simulink subsystem "Day1_Scenario_2"  (R2024a)
settings: Solver=VariableStepAuto  StartTime=0.0  StopTime=10.0  RelTol=1e-3
libraries: CarMaker4SL x2
settings Model: Creator=junhyung.cha  LastModifiedBy=User

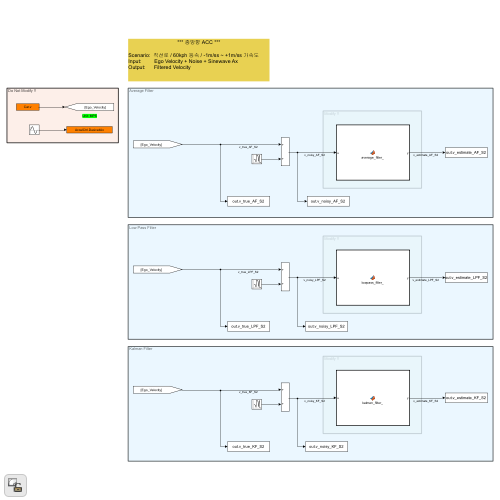
[thumbnail: Simulink's stored preview of the top-level diagram]
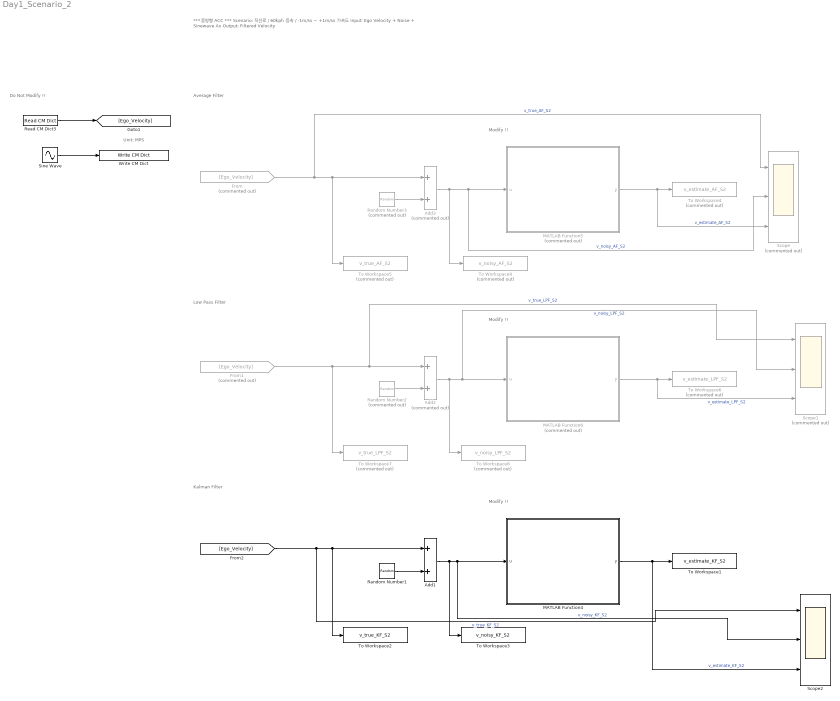
== system Day1_Scenario_2 ==
  note: Do Not Modify !!
  note: Low Pass Filter
  note: Average Filter
  note: Modify !!
  note: Modify !!
  note: Kalman Filter
  note: Modify !!
  note: *** 종방향 ACC ***
      |
      | Scenario: 직선로 / 60kph 등속 / -1m/ss ~ +1m/ss 가속도
      | Input: Ego Velocity + Noise + Sinewave Ax
      | Output: Filtered Velocity
  note: Unit: MPS
  Add1 : Sum
  Add2 : Sum  Commented=on
  Add3 : Sum  Commented=on
  From : From  Commented=on  GotoTag=Ego_Velocity
  From1 : From  Commented=on  GotoTag=Ego_Velocity
  MATLAB Function4 : MATLAB Function  TreatAsAtomicUnit=on
  MATLAB Function5 : MATLAB Function  Commented=on  TreatAsAtomicUnit=on
  MATLAB Function6 : MATLAB Function  Commented=on  TreatAsAtomicUnit=on
  Random Number1 : RandomNumber
  Random Number2 : RandomNumber  Commented=on
  Random Number3 : RandomNumber  Commented=on
  Read CM Dict3 : CarMaker4SL/Read CM Dict  xname=Car.v  xsync=off  xstime=Inherited
  Scope : Scope  Commented=on  NumInputPorts=3
  Scope1 : Scope  Commented=on  NumInputPorts=3
  Scope2 : Scope  NumInputPorts=3
  Sine Wave : Sin
  To Workspace1 : ToWorkspace  VariableName=v_estimate_KF_S2  SaveFormat=Timeseries  SampleTime=-1
  To Workspace2 : ToWorkspace  VariableName=v_true_KF_S2  SaveFormat=Timeseries  SampleTime=-1
  To Workspace3 : ToWorkspace  VariableName=v_noisy_KF_S2  SaveFormat=Timeseries  SampleTime=-1
  To Workspace4 : ToWorkspace  Commented=on  VariableName=v_estimate_AF_S2  SaveFormat=Timeseries  SampleTime=-1
  To Workspace5 : ToWorkspace  Commented=on  VariableName=v_true_AF_S2  SaveFormat=Timeseries  SampleTime=-1
  To Workspace6 : ToWorkspace  Commented=on  VariableName=v_estimate_LPF_S2  SaveFormat=Timeseries  SampleTime=-1
  To Workspace7 : ToWorkspace  Commented=on  VariableName=v_true_LPF_S2  SaveFormat=Timeseries  SampleTime=-1
  To Workspace8 : ToWorkspace  Commented=on  VariableName=v_noisy_LPF_S2  SaveFormat=Timeseries  SampleTime=-1
  To Workspace9 : ToWorkspace  Commented=on  VariableName=v_noisy_AF_S2  SaveFormat=Timeseries  SampleTime=-1
  Write CM Dict : CarMaker4SL/Write CM Dict  xname=AccelCtrl.DesiredAx  xsync=off
  wires:
  Sine Wave/1 -> Write CM Dict/1
  Random Number3/1 -> Add3/2
  Add3/1 -> To Workspace9/1, MATLAB Function5/1(u), Scope/2  "v_noisy_AF_S2"
  Add2/1 -> To Workspace8/1, MATLAB Function6/1(u), Scope1/2  "v_noisy_LPF_S2"
  From1/1 -> Add2/1, Scope1/1, To Workspace7/1  "v_true_LPF_S2"
  MATLAB Function6/1(y) -> To Workspace6/1, Scope1/3  "v_estimate_LPF_S2"
  Random Number2/1 -> Add2/2
  MATLAB Function5/1(y) -> To Workspace4/1, Scope/3  "v_estimate_AF_S2"
  Add1/1 -> To Workspace3/1, MATLAB Function4/1(u), Scope2/2  "v_noisy_KF_S2"
  [Ego_Velocity] -> Add1/1, To Workspace2/1, Scope2/1  "v_true_KF_S2"
  MATLAB Function4/1(y) -> To Workspace1/1, Scope2/3  "v_estimate_KF_S2"
  From/1 -> Add3/1, To Workspace5/1, Scope/1  "v_true_AF_S2"
  Random Number1/1 -> Add1/2
  Read CM Dict3/1 -> [Ego_Velocity]

== matlab function Day1_Scenario_2/MATLAB Function5 ==
  settings: updateMethod=DISCRETE  sampleTime=0.05
  data: u input; y output
% function y = average_filter_(u)
%     y = 0;
% end


function y = average_filter_(u)
% 평균 필터 (5포인트 이동 평균)
% 입력: u - 현재 noisy 값
% 출력: y - 평균 필터된 값

persistent buffer
persistent idx
persistent count

N = 5; % 평균을 낼 샘플 수 (필터 윈도우 크기)

if isempty(buffer)
    buffer = zeros(1, N);
    idx = 1;
    count = 0;
end

% 새로운 값 저장
buffer(idx) = u;
idx = idx + 1;
if idx > N
    idx = 1;
end

% 현재까지 받은 값 수 증가
if count < N
    count = count + 1;
end

% 평균 계산
y = sum(buffer) / count;

== matlab function Day1_Scenario_2/MATLAB Function6 ==
  settings: updateMethod=DISCRETE  sampleTime=0.05
  data: u input; y output
% function y = lowpass_filter_(u)
%     y = 0;
% end

function y = lowpass_filter_(u)
% 1차 로우패스 필터
% 입력: u - 노이즈 포함된 측정값
% 출력: y - 필터링된 추정값

persistent y_prev
persistent alpha

if isempty(y_prev)
    y_prev = 0;     % 출력 초기값
    tau = 0.5;      % 시정수 (조절 가능)
    dt = 0.1;       % 샘플링 시간 (Simulink step time과 맞추세요)
    alpha = dt / (tau + dt);  % 필터 계수 계산
end

% 로우패스 필터 공식
y = alpha * u + (1 - alpha) * y_prev;

% 상태 업데이트
y_prev = y;

== matlab function Day1_Scenario_2/MATLAB Function4 ==
  settings: updateMethod=DISCRETE  sampleTime=0.05
  data: u input; y output
% function y = kalman_filter_(u)
%     y = 0;
% end


function y = kalman_filter_(u)
% u: 측정값 (노이즈 포함된 속도)
% y: 추정된 속도 (칼만 필터 결과)

persistent x_hat P
persistent A H Q R
persistent initialized

if isempty(initialized)
    % 초기 상태
    x_hat = 0;      % 초기 추정값
    P = 1;          % 초기 오차 공분산

    % 시스템 설정
    A = 1;          % 상태 전이 행렬
    H = 1;          % 관측 행렬
    Q = 0.01;       % 프로세스 노이즈 공분산 (시스템의 불확실성)
    R = 0.1;        % 측정 노이즈 공분산 (센서 노이즈 크기)

    initialized = true;
end

% 예측 단계
x_hat_pred = A * x_hat;
P_pred = A * P * A' + Q;

% 칼만 이득 계산
K = P_pred * H' / (H * P_pred * H' + R);

% 업데이트 단계
x_hat = x_hat_pred + K * (u - H * x_hat_pred);
P = (1 - K * H) * P_pred;

% 출력
y = x_hat;
